simulink library "indi_lib"  (R2018b)
settings: Solver=VariableStepAuto  StartTime=0.0  StopTime=10.0  RelTol=1e-3
values from neighbouring files (symbols this model uses):
  G10 = [          inv_I_b * cross( pos, c_XYZ );          c_XYZ / ceb.m      ]    [indiCeFlapFix.m]    (also in indiCePropFix.m = [          2 * inv_I_b * (cep.k*L + cep.d*M .* repmat(cep.a,; indiCopterGetControlEffectiveness.m = 2 * inv(copter.body.I)*(k*L + d*M .* repmat(copter.config.pr)
  G20 = 1 / T_s *      [          inv_I_b * cep.ip * M .* repmat(cep.a,3,1);          zeros( 1, num_motors )      ]    [indiCePropFix.m]    (also in indiCopterGetControlEffectiveness.m = inv(copter.body.I) * copter.prop.I * M .* repmat(copter.conf)
undefined symbols (not defined in the file or in its folder): ca, ceb, cep, DiscIntNeverNeededParam, indiCePropAffineCntrl, mtc, sflt, ts
libraries: ca_lib x2, ndi_lib x2, filters_lib x2, $bdroot x1
settings Model: Creator=Ybeyer  LastModifiedBy=yannic
settings DebuggingCC: LibraryContextMissingDiagnostic=none
settings SFSimCC: SimUseLocalCustomCode=off
settings RTWCC: RTWUseLocalCustomCode=off
settings CodeAppCC: StateflowObjectComments=on

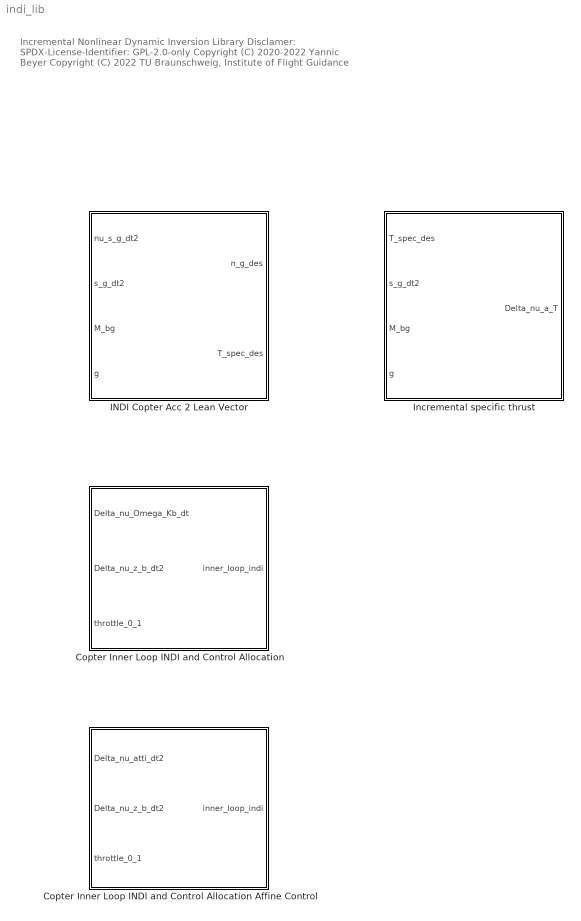
== system indi_lib ==
  note: Incremental Nonlinear Dynamic Inversion Library
      |
      | Disclamer:
      | SPDX-License-Identifier: GPL-2.0-only
      |
      | Copyright (C) 2020-2022 Yannic Beyer
      | Copyright (C) 2022 TU Braunschweig, Institute of Flight Guidance
  Copter Inner Loop INDI and Control Allocation : Subsystem  mask{cep=cep, ceb=ceb, ca=ca, mtc=mtc, sflt=sflt, ts=ts}
      mask prompts: cep "Parameters for motor-propeller control effectiveness, see indiCeProp_params_default"; ceb "Parameters for body control effectiveness, see indiCeBody_params_default"; ca "Control allocation parameters, see controlAllocationWlsLoadParams"; mtc "Motor time constant, s"; sflt "Sensor filter parameters, see indiSensFiltLoadParams"; ts "Sample time, s"
      mask DialogControl DescGroupVar Prompt: Copter Inner Loop INDI and Control Allocation
  Copter Inner Loop INDI and Control Allocation Affine Control : Subsystem  mask{cep=cep, ceb=ceb, ca=ca, mtc=mtc, sflt=sflt, ts=ts}
      mask prompts: cep "Parameters for motor-propeller control effectiveness, see indiCeProp_params_default"; ceb "Parameters for body control effectiveness, see indiCeBody_params_default"; ca "Control allocation parameters, see controlAllocationWlsLoadParams"; mtc "Motor time constant, s"; sflt "Sensor filter parameters, see indiSensFiltLoadParams"; ts "Sample time, s"
      mask init:
      | u_min = ca.u_min;
      | u_max = ca.u_max;
      | u_d = ca.u_d;
      | 
      | U_min = indiCePropAffineCntrl( cep, ca.u_min );
      | U_max = indiCePropAffineCntrl( cep, ca.u_max );
      | U_d = indiCePropAffineCntrl( cep, ca.u_d );
      | 
      | ca.u_min = U_min;
      | ca.u_max = U_max;
      | ca.u_d = U_d;
      mask DialogControl DescGroupVar Prompt: Copter Inner Loop INDI and Control Allocation with Affine Control
      mask DialogControl DescTextVar Prompt: The special feature of this implementation is that the control effectiveness matrix G1 (or renamed G1U here) remains constant, so it does not need to be scheduled. For this purpose, an artificial control input (here called 0 <= U <= 1) was defined, on which the thrust and the torque depend linearly. The actual control input (duty cycle 0 <= u <= 1) is then calculated non-linearly from the artificial control input U.
  INDI Copter Acc 2 Lean Vector : MATLAB Function  TreatAsAtomicUnit=on
  Incremental specific thrust : Subsystem  mask{leanfreq=10, leandamp=1}
      mask prompts: leanfreq "Natural frequency of attitude reference model, rad/s"; leandamp "Damping ratio of attitude reference model"
      mask DialogControl DescGroupVar Prompt: Incremental specific thrust

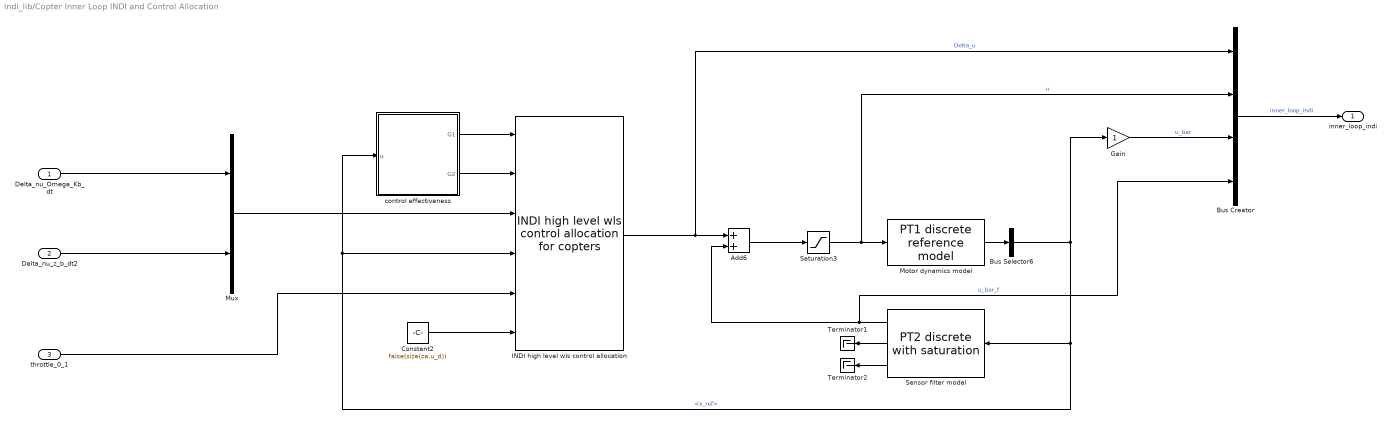
== system indi_lib/Copter Inner Loop INDI and Control Allocation ==
  Delta_nu_Omega_Kb_dt : Inport
  Delta_nu_z_b_dt2 : Inport  Port=2
  throttle_0_1 : Inport  Port=3
  Add6 : Sum
  Bus Creator : BusCreator  Inputs=4
  Bus Selector6 : BusSelector  OutputSignals=x_ref
  Constant2 : Constant  Value=false(size(ca.u_d))
  Gain : Gain
  INDI high level wls control allocation : ca_lib/INDI high level wls control allocation for copters  ca=ca  is_Delta_W_v_check=off  is_W_check=off  is_iter_check=off
  Motor dynamics model : ndi_lib/PT1 discrete reference model  T=mtc  x_max=inf  x_min=-inf  x_dt_max=inf  x_dt_min=-inf  x_init=0
      settings: SourceProductName=LADAC
  Mux : Mux  Inputs=2
  Saturation3 : Saturate  UpperLimit=ca.u_max  LowerLimit=ca.u_min
  Sensor filter model : filters_lib/PT2 discrete with saturation  param_src=internal  omega=sflt.omega  d=sflt.D  x_dt2_max=inf  x_dt2_min=-inf  x_dt_max=inf  x_dt_min=-inf  x_max=inf  x_min=-inf  y_0_src=internal  x_init=0  y_dt_0_src=internal  x_dt_init=0  is_y_dt_checked=on  is_y_dt2_checked=on
      settings: SourceProductName=LADAC
  Terminator1 : Terminator
  Terminator2 : Terminator
  control effectiveness : Subsystem  mask{cep=cep, ceb=ceb, ts=ts, u_min=ca.u_min}
      mask prompts: cep "propeller control effectiveness struct, see cntrlEffectPropLoadParams"; ceb "body control effectiveness struct, see cntrlEffectBodyLoadParams"; ts "controller sample time, s"
      mask init:
      | [G10,G20] = indiCePropFix( cep, ceb, ts );
  inner_loop_indi : Outport
  wires:
  Sensor filter model/1 -> Add6/2, Bus Creator/4  "u_bar_f"
  Mux/1 -> INDI high level wls control allocation/3
  Saturation3/1 -> Bus Creator/2, Motor dynamics model/1  "u"
  INDI high level wls control allocation/1 -> Bus Creator/1, Add6/1  "Delta_u"
  throttle_0_1/1 -> INDI high level wls control allocation/5
  Bus Selector6/1 -> Gain/1, Sensor filter model/1, control effectiveness/1(u), INDI high level wls control allocation/4  "<x_ref>"
  control effectiveness/1(G1) -> INDI high level wls control allocation/1
  Constant2/1 -> INDI high level wls control allocation/6
  Sensor filter model/2 -> Terminator1/1
  Sensor filter model/3 -> Terminator2/1
  Motor dynamics model/1 -> Bus Selector6/1
  Add6/1 -> Saturation3/1
  Delta_nu_Omega_Kb_dt/1 -> Mux/1
  control effectiveness/2(G2) -> INDI high level wls control allocation/2
  Delta_nu_z_b_dt2/1 -> Mux/2
  Gain/1 -> Bus Creator/3  "u_bar"
  Bus Creator/1 -> inner_loop_indi/1  "inner_loop_indi"

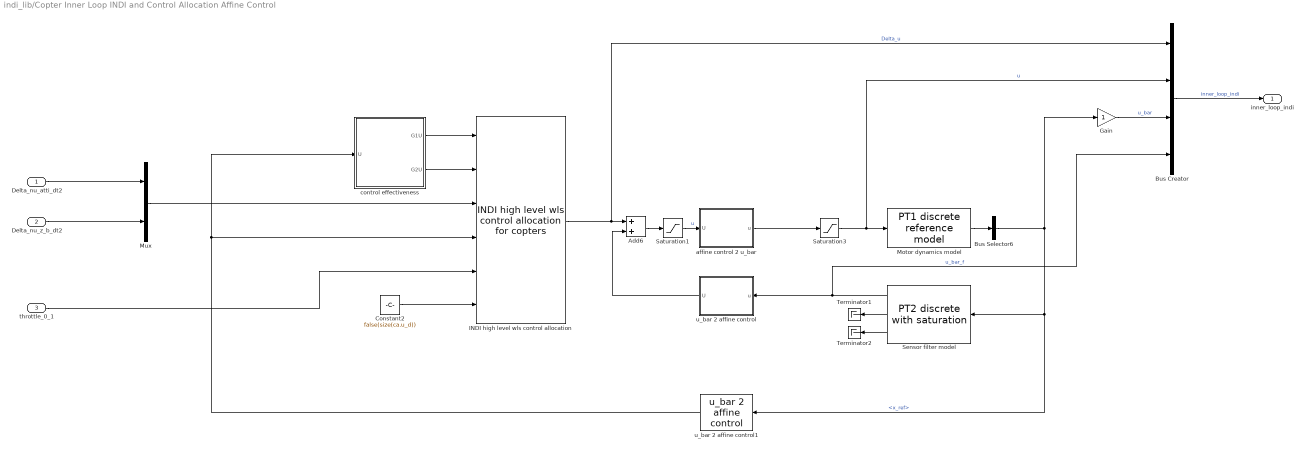
== system indi_lib/Copter Inner Loop INDI and Control Allocation Affine Control ==
  Delta_nu_atti_dt2 : Inport
  Delta_nu_z_b_dt2 : Inport  Port=2
  throttle_0_1 : Inport  Port=3
  Add6 : Sum
  Bus Creator : BusCreator  Inputs=4
  Bus Selector6 : BusSelector  OutputSignals=x_ref
  Constant2 : Constant  Value=false(size(ca.u_d))
  Gain : Gain
  INDI high level wls control allocation : ca_lib/INDI high level wls control allocation for copters  ca=ca  is_Delta_W_v_check=off  is_W_check=off  is_iter_check=off
  Motor dynamics model : ndi_lib/PT1 discrete reference model  T=mtc  x_max=inf  x_min=-inf  x_dt_max=inf  x_dt_min=-inf  x_init=0
      settings: SourceProductName=LADAC
  Mux : Mux  Inputs=2
  Saturation1 : Saturate  UpperLimit=indiCePropAffineCntrl( cep, ca.u_max )  LowerLimit=indiCePropAffineCntrl( cep, ca.u_min )
  Saturation3 : Saturate  UpperLimit=u_max  LowerLimit=u_min
  Sensor filter model : filters_lib/PT2 discrete with saturation  param_src=internal  omega=sflt.omega  d=sflt.D  x_dt2_max=inf  x_dt2_min=-inf  x_dt_max=inf  x_dt_min=-inf  x_max=inf  x_min=-inf  y_0_src=internal  x_init=0  y_dt_0_src=internal  x_dt_init=0  is_y_dt_checked=on  is_y_dt2_checked=on
      settings: SourceProductName=LADAC
  Terminator1 : Terminator
  Terminator2 : Terminator
  affine control 2 u_bar : Subsystem  mask{cep=cep}
  control effectiveness : Subsystem  mask{cep=cep, ceb=ceb, ts=ts, u_min=ca.u_min}
      mask prompts: cep "propeller control effectiveness struct, see cntrlEffectPropLoadParams"; ceb "body control effectiveness struct, see cntrlEffectBodyLoadParams"; ts "controller sample time, s"
      mask init:
      | [G10,G20] = indiCePropFix( cep, ceb, ts );
      | 
      | u_max = ones(4,1);
      | 
      | omega_max = motorStaticSpeed( cep.kt, cep.ri, cep.vb, cep.d, u_max );
      | omega2 = diag( omega_max.^2 );
      | 
      | G1U = 0.5 * G10 * omega2;
  u_bar 2 affine control : Subsystem  mask{cep=cep}
  u_bar 2 affine control1 : $bdroot/Copter Inner Loop INDI and Control Allocation Affine Control/u_bar 2 affine control  cep=cep
  inner_loop_indi : Outport
  wires:
  throttle_0_1/1 -> INDI high level wls control allocation/5
  Sensor filter model/1 -> Bus Creator/4, u_bar 2 affine control/1(u)  "u_bar_f"
  Sensor filter model/2 -> Terminator1/1
  Add6/1 -> Saturation1/1
  INDI high level wls control allocation/1 -> Bus Creator/1, Add6/1  "Delta_u"
  affine control 2 u_bar/1(u) -> Saturation3/1
  Motor dynamics model/1 -> Bus Selector6/1
  Constant2/1 -> INDI high level wls control allocation/6
  Sensor filter model/3 -> Terminator2/1
  Delta_nu_atti_dt2/1 -> Mux/1
  Saturation3/1 -> Bus Creator/2, Motor dynamics model/1  "u"
  u_bar 2 affine control1/1 -> control effectiveness/1(U), INDI high level wls control allocation/4
  Bus Selector6/1 -> Gain/1, u_bar 2 affine control1/1, Sensor filter model/1  "<x_ref>"
  Delta_nu_z_b_dt2/1 -> Mux/2
  Saturation1/1 -> affine control 2 u_bar/1(U)  "u"
  Mux/1 -> INDI high level wls control allocation/3
  u_bar 2 affine control/1(U) -> Add6/2
  control effectiveness/1(G1U) -> INDI high level wls control allocation/1
  control effectiveness/2(G2U) -> INDI high level wls control allocation/2
  Bus Creator/1 -> inner_loop_indi/1  "inner_loop_indi"
  Gain/1 -> Bus Creator/3  "u_bar"

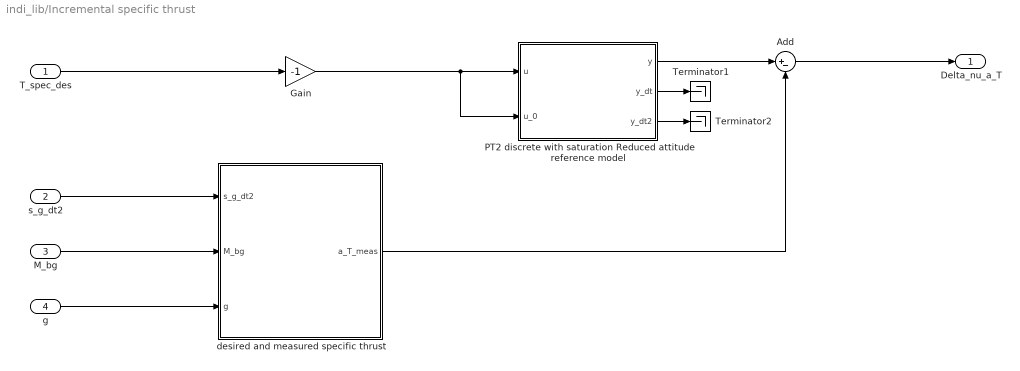
== system indi_lib/Incremental specific thrust ==
  T_spec_des : Inport
  s_g_dt2 : Inport  Port=2
  M_bg : Inport  Port=3
  g : Inport  Port=4
  Add : Sum  Inputs=|+-
  Gain : Gain  Gain=-1
  PT2 discrete with saturation Reduced attitude reference model : Subsystem  mask{omega=leanfreq, d=leandamp, x_dt2_max=inf, x_dt2_min=-inf, x_dt_max=inf, x_dt_min=-inf, x_max=inf, x_min=-inf, x_init=0, x_dt_init=0}
      mask prompts: omega "Natural frequency"; d "Damping ratio"; x_dt2_max "Maximum acceleration"; x_dt2_min "Minimum acceleration"; x_dt_max "Maximum rate"; x_dt_min "Minimum rate"; x_max "Maximum position"; x_min "Minimum position"; x_init "Initial position"; x_dt_init "Initial rate"
  Terminator1 : Terminator
  Terminator2 : Terminator
  desired and measured specific thrust : MATLAB Function  TreatAsAtomicUnit=on
  Delta_nu_a_T : Outport
  wires:
  PT2 discrete with saturation Reduced attitude reference model/2(y_dt) -> Terminator1/1
  PT2 discrete with saturation Reduced attitude reference model/3(y_dt2) -> Terminator2/1
  PT2 discrete with saturation Reduced attitude reference model/1(y) -> Add/1
  T_spec_des/1 -> Gain/1
  desired and measured specific thrust/1(a_T_meas) -> Add/2
  Add/1 -> Delta_nu_a_T/1
  s_g_dt2/1 -> desired and measured specific thrust/1(s_g_dt2)
  M_bg/1 -> desired and measured specific thrust/2(M_bg)
  g/1 -> desired and measured specific thrust/3(g)
  Gain/1 -> PT2 discrete with saturation Reduced attitude reference model/2(u_0), PT2 discrete with saturation Reduced attitude reference model/1(u)

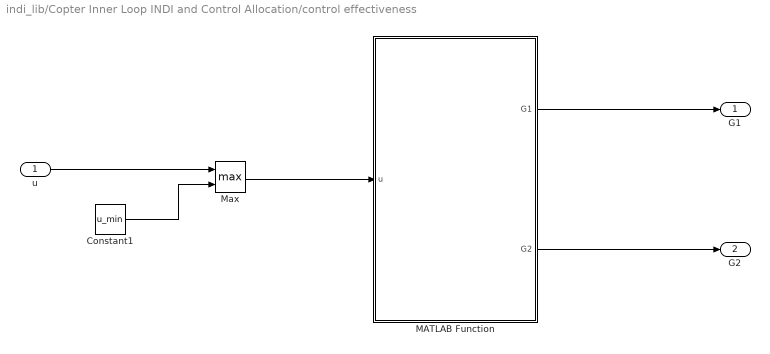
== system indi_lib/Copter Inner Loop INDI and Control Allocation/control effectiveness ==
  u : Inport
  Constant1 : Constant  Value=u_min
  MATLAB Function : MATLAB Function  TreatAsAtomicUnit=on
  Max : MinMax  Function=max  Inputs=2  OutDataTypeStr=Inherit: Inherit via back propagation
  G1 : Outport
  G2 : Outport  Port=2
  wires:
  u/1 -> Max/1
  Constant1/1 -> Max/2
  Max/1 -> MATLAB Function/1(u)
  MATLAB Function/1(G1) -> G1/1
  MATLAB Function/2(G2) -> G2/1

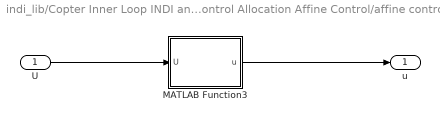
== system indi_lib/Copter Inner Loop INDI and Control Allocation Affine Control/affine control 2 u_bar ==
  U : Inport
  MATLAB Function3 : MATLAB Function  TreatAsAtomicUnit=on
  u : Outport
  wires:
  MATLAB Function3/1(u) -> u/1
  U/1 -> MATLAB Function3/1(U)

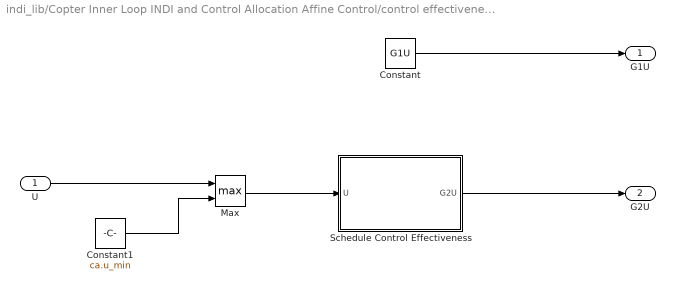
== system indi_lib/Copter Inner Loop INDI and Control Allocation Affine Control/control effectiveness ==
  U : Inport
  Constant : Constant  Value=G1U
  Constant1 : Constant  Value=ca.u_min
  Max : MinMax  Function=max  Inputs=2  OutDataTypeStr=Inherit: Inherit via back propagation
  Schedule Control Effectiveness : MATLAB Function  TreatAsAtomicUnit=on
  G1U : Outport
  G2U : Outport  Port=2
  wires:
  U/1 -> Max/1
  Constant1/1 -> Max/2
  Max/1 -> Schedule Control Effectiveness/1(U)
  Schedule Control Effectiveness/1(G2U) -> G2U/1
  Constant/1 -> G1U/1

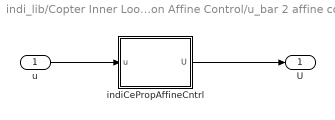
== system indi_lib/Copter Inner Loop INDI and Control Allocation Affine Control/u_bar 2 affine control ==
  u : Inport
  indiCePropAffineCntrl : MATLAB Function  TreatAsAtomicUnit=on
  U : Outport
  wires:
  u/1 -> indiCePropAffineCntrl/1(u)
  indiCePropAffineCntrl/1(U) -> U/1

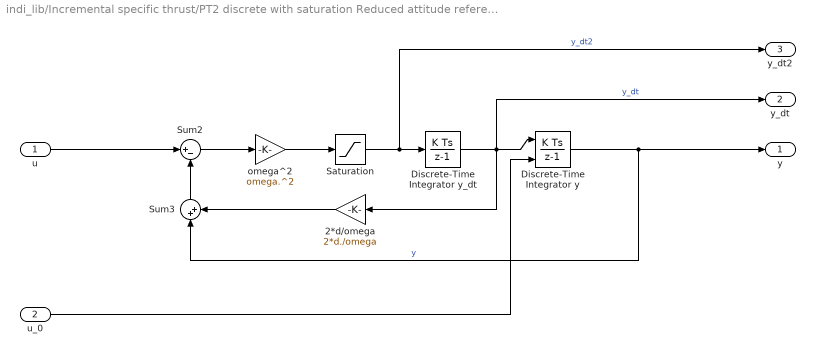
== system indi_lib/Incremental specific thrust/PT2 discrete with saturation Reduced attitude reference model ==
  u : Inport
  u_0 : Inport  Port=2
  2*d/omega : Gain  Gain=2*d./omega
  Discrete-Time Integrator y : DiscreteIntegrator  InitialConditionSource=external  InitialCondition=x_init  SampleTime=-1  OutDataTypeStr=Inherit: Inherit via back propagation  LimitOutput=on  UpperSaturationLimit=x_max  LowerSaturationLimit=x_min  ICPrevOutput=DiscIntNeverNeededParam  ICPrevScaledInput=DiscIntNeverNeededParam
  Discrete-Time Integrator y_dt : DiscreteIntegrator  InitialCondition=x_dt_init  SampleTime=-1  OutDataTypeStr=Inherit: Inherit via back propagation  LimitOutput=on  UpperSaturationLimit=x_dt_max  LowerSaturationLimit=x_dt_min  ICPrevOutput=DiscIntNeverNeededParam  ICPrevScaledInput=DiscIntNeverNeededParam
  Saturation : Saturate  UpperLimit=x_dt2_max  LowerLimit=x_dt2_min
  Sum2 : Sum  Inputs=|+-
  Sum3 : Sum  Inputs=|++
  omega^2 : Gain  Gain=omega.^2
  y : Outport
  y_dt : Outport  Port=2
  y_dt2 : Outport  Port=3
  wires:
  u_0/1 -> Discrete-Time Integrator y/2
  Discrete-Time Integrator y_dt/1 -> Discrete-Time Integrator y/1, y_dt/1, 2*d/omega/1  "y_dt"
  Discrete-Time Integrator y/1 -> y/1, Sum3/1  "y"
  Sum2/1 -> omega^2/1
  2*d/omega/1 -> Sum3/2
  u/1 -> Sum2/1
  Sum3/1 -> Sum2/2
  omega^2/1 -> Saturation/1
  Saturation/1 -> Discrete-Time Integrator y_dt/1, y_dt2/1  "y_dt2"

== matlab function indi_lib/Copter Inner Loop INDI and Control Allocation/control effectiveness/MATLAB Function ==
  data: cep parameter; G10 parameter; G20 parameter; u input; G1 output; G2 output
function [G1,G2] = indiCePropVar( cep, G10, G20, u ) %#codegen
[G1,G2] = indiCePropVar( cep, G10, G20, u );
end

== matlab function indi_lib/INDI Copter Acc 2 Lean Vector ==
  data: nu_s_g_dt2 input; n_g_des output; s_g_dt2 input; M_bg input; g input; T_spec_des output
function [n_g_des,T_spec_des] = indiCopterAcc2LeanVector( nu_s_g_dt2, s_g_dt2, M_bg, g )
[n_g_des,T_spec_des] = indiCopterAcc2LeanVector( nu_s_g_dt2, s_g_dt2, M_bg, g );
end

== matlab function indi_lib/Copter Inner Loop INDI and Control Allocation Affine Control/control effectiveness/Schedule Control Effectiveness ==
  data: G20 parameter; omega_max parameter; U input; G2U output
function G2U = fcn( G20, omega_max, U ) %#codegen

omega_dU = diag( divideFinite( omega_max/2, sqrtReal( U ) ) );

G2U = G20 * omega_dU;

end

== matlab function indi_lib/Copter Inner Loop INDI and Control Allocation Affine Control/u_bar 2 affine control/indiCePropAffineCntrl ==
  data: u input; U output; cep parameter
function U = fcn(u,cep)
U = indiCePropAffineCntrl( cep, u );
end

== matlab function indi_lib/Copter Inner Loop INDI and Control Allocation Affine Control/affine control 2 u_bar/MATLAB Function3 ==
  data: U input; u output; cep parameter
function u = fcn(U,cep)

% u = ((2^(1/2)*(cep.kt*U*(cep.kt^3 - cep.kt*(cep.kt^4 + 4*cep.ri*cep.vb*cep.d*cep.kt)^(1/2) ...
%     + 2*cep.ri*cep.vb*cep.d)).^(1/2) - cep.kt^2).^2 - cep.kt^4)/(4*cep.kt*cep.ri*cep.vb*cep.d);
% u = ((U*((cep.kt^4 + 4*cep.ri*cep.vb*cep.d*cep.kt)^(1/2) - cep.kt^2) + cep.kt^2).^2 - cep.kt^4)./(4*cep.kt*cep.ri*cep.vb*cep.d);
u = -(cep.kt^4 - (2^(1/2)*(cep.kt*U*(cep.kt^3 - cep.kt*(cep.kt^4 + 4*cep.ri*cep.vb*cep.d*cep.kt)^(1/2) ...
    + 2*cep.ri*cep.vb*cep.d)).^(1/2) + cep.kt^2).^2)./(4*cep.kt*cep.ri*cep.vb*cep.d);

end

== matlab function indi_lib/Incremental specific thrust/desired and measured specific thrust ==
  data: s_g_dt2 input; a_T_meas output; M_bg input; g input
function a_T_meas = fcn(s_g_dt2,M_bg, g)

a_b_meas = M_bg * s_g_dt2;

g_g = [0;0;g];
g_b = M_bg * g_g;
a_T_meas = a_b_meas(3) - g_b(3);

end
